simulink model "ventilation_system"  (R2021a)
settings: Solver=VariableStepAuto  StartTime=0.0  StopTime=2.6e6  RelTol=1e-3
model workspace (MAT data in the model file):
  door_area = 1.2
  duct_area = 0.01
  zone_flow_area = 10.9375
undefined symbols (not defined in the file): initial_temperature
libraries: nesl_utility x3, fl_lib x2
settings Model: OrderedModelArguments=off  Creator=Michael.Mittermaier  LastModifiedBy=mm
settings SolverCC: AlgebraicLoopSolver=TrustRegion
settings DebuggingCC: SFMachineParentedDataDiag=warning

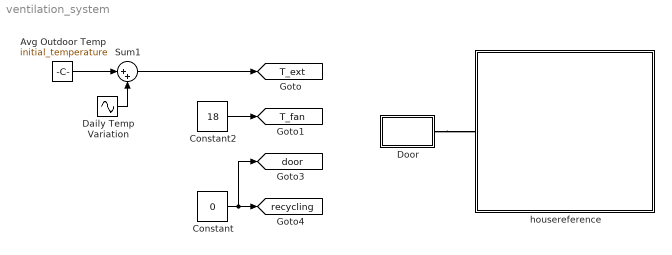
== system ventilation_system ==
  Avg Outdoor Temp : Constant  Value=initial_temperature
  Constant : Constant  Value=0
  Constant2 : Constant  Value=18
  Daily Temp Variation : Sin  Amplitude=5  Frequency=2*pi/86400  SampleTime=0
  Door : Subsystem
  Sum1 : Sum  Inputs=|++  InputSameDT=on  SaturateOnIntegerOverflow=on  OutDataTypeStr=Inherit: Same as first input
  housereference : Subsystem  ReferencedSubsystem=house0000_subsys
  tag scope: T_ext=global, T_fan=global, door=global, recycling=global
  wires:
  Avg Outdoor Temp/1 -> Sum1/1
  Sum1/1 -> [T_ext]
  Constant/1 -> [door], [recycling]
  Constant2/1 -> [T_fan]
  Daily Temp Variation/1 -> Sum1/2
  connections:
  Door/RConn1 -- housereference/LConn1

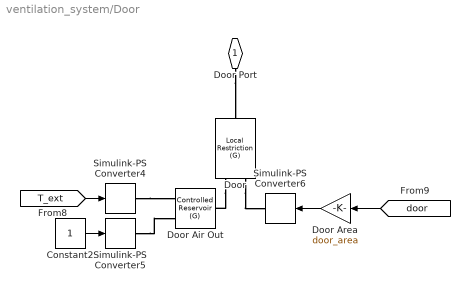
== system ventilation_system/Door ==
  Constant2 : Constant
  Door : fl_lib/Gas/Elements/Local Restriction (G)  restriction_type=foundation.enum.restriction_type.variable  restriction_area=1e-3 m^2  min_area=1e-10 m^2  max_area=0.5*door_area m^2  area=door_area m^2  Cd=0.8  B_lam=0.999
      settings: SourceProductBaseCode=SS  InternalSimscapePortConfiguration="{\"Bottom\":[],\"Left\":[{\"id\":\"A\",\"label\":\"A\",\"type\":\"foundation.gas.gas\"},{\"id\":\"area_in\",\"label\":\"AR\",\"type\":\"input\"}],\"Right\":[{\"id\":\"B\",\"label\":\"B\",\"type\":\"foundation.gas.gas\"}],\"Top\":[]}"
  Door Air Out : fl_lib/Gas/Elements/Controlled Reservoir (G)  area_A=door_area m^2
      settings: SourceProductName=Foundation Library  InternalSimscapePortConfiguration="{\"Bottom\":[],\"Left\":[{\"id\":\"A\",\"label\":\"A\",\"type\":\"foundation.gas.gas\"}],\"Right\":[{\"id\":\"T_in\",\"label\":\"T\",\"type\":\"input\"},{\"id\":\"p_in\",\"label\":\"P\",\"type\":\"input\"}],\"Top\":[]}"
  Door Area : Gain  Gain=door_area
  Simulink-PS Converter4 : nesl_utility/Simulink-PS Converter  PhysicalDomain=network_engine_domain  SubClassName=ps_input  LeftPortType=input  RightPortType=output  PseudoPeriodic=off  Frequencies=[]  NoiseDistribution=none  NoiseParameters=[]  Unit=degC  AffineConversion=on  FilteringAndDerivatives=provide  SimscapeFilterOrder=1  InputFilterTimeConstant=0.001  UdotUserProvided=0
      settings: SourceProductBaseCode=PW,SS
  Simulink-PS Converter5 : nesl_utility/Simulink-PS Converter  PhysicalDomain=network_engine_domain  SubClassName=ps_input  LeftPortType=input  RightPortType=output  PseudoPeriodic=off  Frequencies=[]  NoiseDistribution=none  NoiseParameters=[]  Unit=atm  AffineConversion=off  FilteringAndDerivatives=provide  SimscapeFilterOrder=1  InputFilterTimeConstant=0.001  UdotUserProvided=0
      settings: SourceProductBaseCode=PW,SS
  Simulink-PS Converter6 : nesl_utility/Simulink-PS Converter  PhysicalDomain=network_engine_domain  SubClassName=ps_input  LeftPortType=input  RightPortType=output  PseudoPeriodic=off  Frequencies=[]  NoiseDistribution=none  NoiseParameters=[]  Unit=m^2  AffineConversion=off  FilteringAndDerivatives=provide  SimscapeFilterOrder=1  InputFilterTimeConstant=0.001  UdotUserProvided=0
      settings: SourceProductBaseCode=PW,SS
  Door Port : PMIOPort  Side=Right
  wires:
  Constant2/1 -> Simulink-PS Converter5/1
  [T_ext] -> Simulink-PS Converter4/1
  [door] -> Door Area/1
  Door Area/1 -> Simulink-PS Converter6/1
  connections:
  Simulink-PS Converter5/RConn1 -- Door Air Out/RConn2
  Simulink-PS Converter4/RConn1 -- Door Air Out/RConn1
  Door/LConn1 -- Door Air Out/LConn1
  Door/LConn2 -- Simulink-PS Converter6/RConn1
  Door Port/RConn1 -- Door/RConn1
